simulink model "A03_L10_2"  (R2021b)
settings: Solver=ode45  StartTime=0.0  StopTime=5  RelTol=1e-3  EnableMultiTasking=on
values from neighbouring files (symbols this model uses):
  h = 0.1    [A04_L10_script.m]
  k1d = 0.01    [A04_L10_script.m]
  k2d = -0.18    [A04_L10_script.m]
  kwd = 1    [A04_L10_script.m]
libraries: simulink x1
settings Model: Creator=User  LastModifiedBy=Adi
settings SolverCC: AlgebraicLoopSolver=TrustRegion
settings DataIOCC: LimitDataPoints=on  SaveFormat=Array  ReturnWorkspaceOutputs=off
settings OptimizationCC: LifeSpan=inf
settings DebuggingCC: SolverPrmCheckMsg=warning  SFUnexpectedBacktrackingDiag=warning  SFNoUnconditionalDefaultTransitionDiag=warning  SFExecutionAtInitializationDiag=none  SFMachineParentedDataDiag=warning  ArithmeticOperatorsInVariantConditions=warning
settings HardwareCC: ProdBitPerPointer=32  ProdBitPerSizeT=32  ProdBitPerPtrDiffT=32  ProdLargestAtomicFloat=None  ProdIntDivRoundTo=Undefined  ProdEndianess=Unspecified  ProdWordSize=32  ProdHWDeviceType=32-bit Generic
settings ModelReferenceCC: PropagateSignalLabelsOutOfModel=off
settings SFSimCC: SimUseLocalCustomCode=off  CustomCodeUndefinedFunction=UseInterfaceOnly
settings RTWCC: RTWUseLocalCustomCode=off
settings CodeAppCC: StateflowObjectComments=on
settings GRTTargetCC: TargetLangStandard=C89/C90 (ANSI)
settings ConfigComp: CovMetricSettings=dw  CovSaveCumulativeToWorkspaceVar=on  CovSaveSingleToWorkspaceVar=on  CovExternalEMLEnable=off  CovSFcnEnable=off

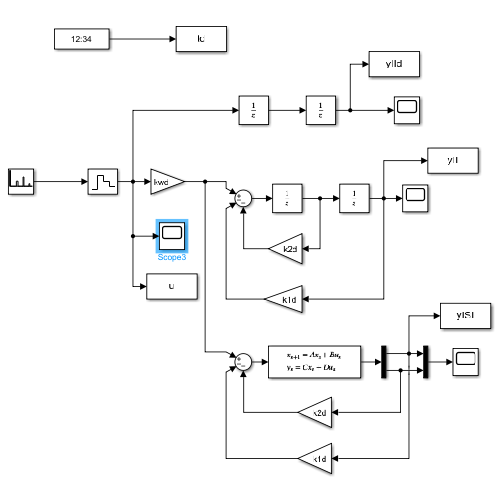
[thumbnail: Simulink's stored preview of the top-level diagram]
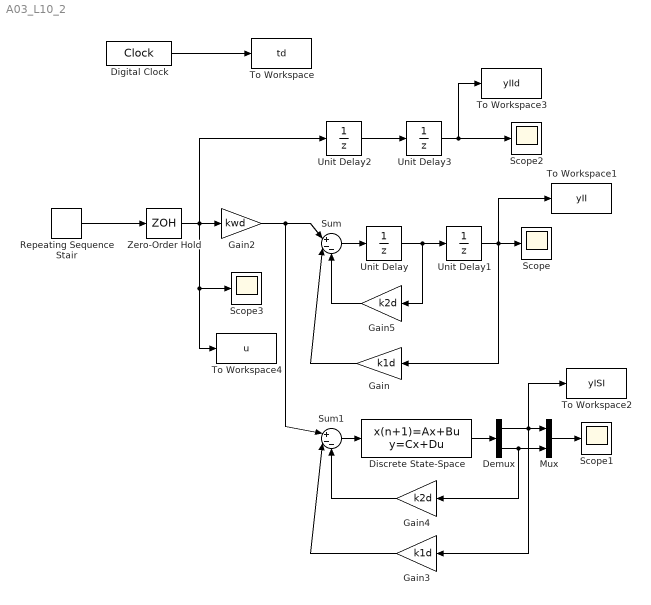
== system A03_L10_2 ==
  Demux : Demux  Outputs=2
  Digital Clock : DigitalClock  SampleTime=0.01
  Discrete State-Space : DiscreteStateSpace  A=[0 1;0 0]  B=[0;1]  C=[1 0;0 1]  D=[0;0]  InitialCondition=[0;0]  SampleTime=h
  Gain : Gain  Gain=k1d  SampleTime=h
  Gain2 : Gain  Gain=kwd  SampleTime=h
  Gain3 : Gain  Gain=k1d  SampleTime=h
  Gain4 : Gain  Gain=k2d  SampleTime=h
  Gain5 : Gain  Gain=k2d  SampleTime=h
  Mux : Mux  Inputs=2
  Repeating Sequence Stair : simulink/Sources/Repeating Sequence Stair  OutValues="[3 0 0 0 0 0 1 0 0  0 0 1.8 0 0 0 0 0.5 0 0]'"  tsamp=h  OutMin=[]  OutMax=[]  OutDataTypeStr=double  OutputDataTypeScalingMode=double  OutDataType=fixdt(0,8)  ConRadixGroup=Best Precision: Vector-wise  OutScaling=2^-12
  Scope{,1..3} (4 alike) : Scope
  Sum : Sum  Inputs=|+--
  Sum1 : Sum  Inputs=|+--
  To Workspace : ToWorkspace  VariableName=td  SampleTime=h
  To Workspace1 : ToWorkspace  VariableName=yII  SampleTime=h
  To Workspace2 : ToWorkspace  VariableName=yISI  SampleTime=h
  To Workspace3 : ToWorkspace  VariableName=yIId  SampleTime=h
  To Workspace4 : ToWorkspace  VariableName=u  SampleTime=h
  Unit Delay{,1..3} (4 alike) : UnitDelay  SampleTime=h  HasFrameUpgradeWarning=on
  Zero-Order Hold : ZeroOrderHold  SampleTime=h
  wires:
  Unit Delay/1 -> Unit Delay1/1, Gain5/1
  Sum/1 -> Unit Delay/1
  Digital Clock/1 -> To Workspace/1
  Gain5/1 -> Sum/3
  Gain/1 -> Sum/2
  Sum1/1 -> Discrete State-Space/1
  Zero-Order Hold/1 -> Scope3/1, To Workspace4/1, Unit Delay2/1, Gain2/1
  Gain4/1 -> Sum1/3
  Gain3/1 -> Sum1/2
  Discrete State-Space/1 -> Demux/1
  Demux/1 -> To Workspace2/1, Gain3/1, Mux/1
  Demux/2 -> Gain4/1, Mux/2
  Mux/1 -> Scope1/1
  Unit Delay1/1 -> To Workspace1/1, Gain/1, Scope/1
  Unit Delay2/1 -> Unit Delay3/1
  Gain2/1 -> Sum1/1, Sum/1
  Unit Delay3/1 -> Scope2/1, To Workspace3/1
  Repeating Sequence Stair/1 -> Zero-Order Hold/1
